simulink model "linearized_EOM"  (R2020a)
settings: Solver=VariableStepAuto  StartTime=0.0  StopTime=10.0  RelTol=1e-3
values from neighbouring files (symbols this model uses):
  Beq = 5.4    [setup_ip01_2_configuration.m]
  Eff_g = 1    [setup_ip01_2_configuration.m]
  Eff_m = 1    [setup_ip01_2_configuration.m]
  Kg = 3.71    [setup_ip01_2_configuration.m]
  Km = 0.804e-3 * K_RDPS2RPM    [setup_ip01_2_configuration.m]
  Kt = 1.088 * K_OZ2N * K_IN2M    [setup_ip01_2_configuration.m]
  Mc = Mc + Eff_g * Kg^2 * Jm / r_mp^2    [setup_lab_ip02_spg.m]
  r_mp = 0.5 / 2 * K_IN2M    [setup_ip01_2_configuration.m]
  Rm = 2.6    [setup_ip01_2_configuration.m]
undefined symbols (not defined in the file or in its folder): Bp, g, Ip, lp, Mp
settings Model: Creator=Tomo  LastModifiedBy=Tomo

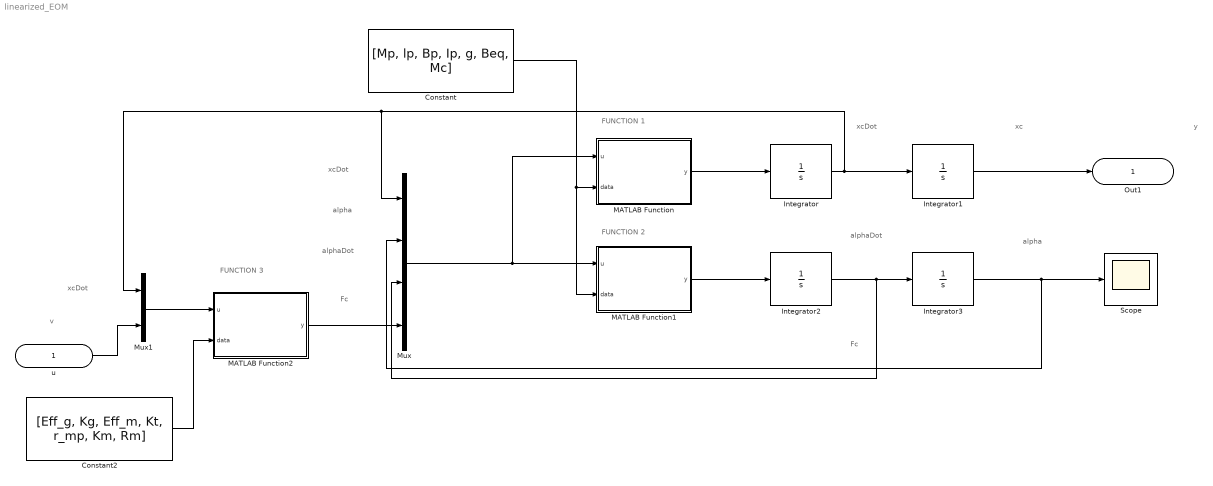
== system linearized_EOM ==
  note: FUNCTION 1
  note: v
  note: Fc
  note: alphaDot
  note: alpha
  note: xc
  note: xcDot
  note: xcDot
  note: alpha
  note: alphaDot
  note: Fc
  note: y
  note: FUNCTION 2
  note: FUNCTION 3
  note: xcDot
  u : Inport
  Constant : Constant  Value=[Mp, lp, Bp, Ip, g, Beq, Mc]  VectorParams1D=off
  Constant2 : Constant  Value=[Eff_g, Kg, Eff_m, Kt, r_mp, Km, Rm]  VectorParams1D=off
  Integrator : Integrator
  Integrator1 : Integrator
  Integrator2 : Integrator  InitialCondition=pi/2
  Integrator3 : Integrator
  MATLAB Function : MATLAB Function  TreatAsAtomicUnit=on
  MATLAB Function1 : MATLAB Function  TreatAsAtomicUnit=on
  MATLAB Function2 : MATLAB Function  TreatAsAtomicUnit=on
  Mux : Mux
  Mux1 : Mux  Inputs=2
  Scope : Scope
  Out1 : Outport
  wires:
  Mux/1 -> MATLAB Function/1(u), MATLAB Function1/1(u)
  MATLAB Function1/1(y) -> Integrator2/1
  Integrator2/1 -> Mux/3, Integrator3/1
  MATLAB Function/1(y) -> Integrator/1
  Integrator/1 -> Integrator1/1, Mux1/1, Mux/1
  Integrator1/1 -> Out1/1
  Integrator3/1 -> Mux/2, Scope/1
  Constant/1 -> MATLAB Function1/2(data), MATLAB Function/2(data)
  MATLAB Function2/1(y) -> Mux/4
  Constant2/1 -> MATLAB Function2/2(data)
  u/1 -> Mux1/2
  Mux1/1 -> MATLAB Function2/1(u)

== matlab function linearized_EOM/MATLAB Function ==
  data: u input size=4; y output; data input size=7
function y = fcn(u, data)
    % FUNCTION 1
    Mp = data(1); lp = data(2); Bp = data(3); Ip = data(4); g = data(5);
    Beq = data(6); Mc = data(7); 
    xcdot = u(1); a = u(2); adot = u(3); Fc = u(4);
    
    den = (Mc + Mp)*Ip + Mc*Mp*lp^2 + Mp^2*lp^2*sin(a)^2;
    num1 = Mp*lp*Bp*cos(a)*adot;
    num2 = (Mp^2*lp^3 + Ip*Mp*lp)*sin(a)*adot^2;
    num3 = (Ip + Mp*lp^2)*Fc;
    num4 = Mp^2*lp^2*g*cos(a)*sin(a);
    num5 = -(Ip + Mp*lp^2)*Beq*xcdot;
    
    y = (num1 + num2 + num3 + num4 + num5) / den;
end

== matlab function linearized_EOM/MATLAB Function2 ==
  data: u input size=2; y output; data input size=7
function y = fcn(u, data)
    % FUNCTION 3
    Eff_g = data(1); Kg = data(2); 
    Eff_m = data(3); Kt = data(4); r_mp = data(5); 
    Km = data(6); Rm = data(7); 
    xcdot = u(1); v = u(2);
    
    den = Rm*r_mp^2;
    num = Eff_g*Kg*Eff_m*Kt * (v*r_mp - Kg*Km*xcdot);
    
    y = num / den;
end

== matlab function linearized_EOM/MATLAB Function1 ==
  data: u input size=4; y output; data input size=7
function y = fcn(u, data)
    % FUNCTION 2
    Mp = data(1); lp = data(2); Bp = data(3); Ip = data(4); g = data(5);
    Beq = data(6); Mc = data(7);
    xcdot = u(1); a = u(2); adot = u(3); Fc = u(4);
    
    den = (Mc + Mp)*Ip + Mc*Mp*lp^2 + Mp^2*lp^2*sin(a)^2;
    num1 = Mp*lp*cos(a)*Beq*xcdot;
    num2 = -(Mc + Mp)*Mp*g*lp*sin(a);
    num3 = -Mp^2*lp^2*sin(a)*cos(a)*adot^2;
    num4 = -Mp*lp*cos(a)*Fc;
    num5 = -(Mc + Mp)*Bp*adot;
    
    y = (num1 + num2 + num3 + num4 + num5) / den;
end
